simulink model "SystemSimulation"  (R2022a)
settings: Solver=VariableStepAuto  StartTime=0.0  StopTime=Tsim  RelTol=1e-3
values from neighbouring files (symbols this model uses):
  b = 0.0686    [epsac_elbow.m]    (also in modelFinder.m)
  g = 0.8234    [epsac_elbow.m]    (also in modelFinder.m)
  h = 0.3632    [epsac_elbow.m]    (also in modelFinder.m)
  Jeq = 5.4579e-4    (= 0.00054579)    [epsac_elbow.m]    (also in modelFinder.m)
  k = -0.0056    [epsac_elbow.m]    (also in modelFinder.m)
  M = 0.0857    [epsac_elbow.m]    (also in modelFinder.m)
  m = 0.2853    [epsac_elbow.m]    (also in modelFinder.m)
  x = x - x(1)    [modelFinder.m]
settings Model: Creator=aaron  LastModifiedBy=aaron

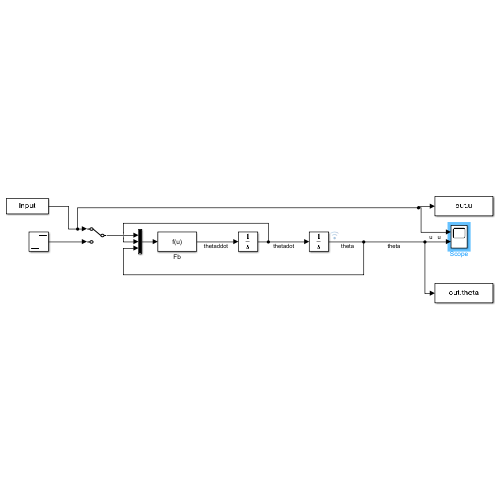
[thumbnail: Simulink's stored preview of the top-level diagram]
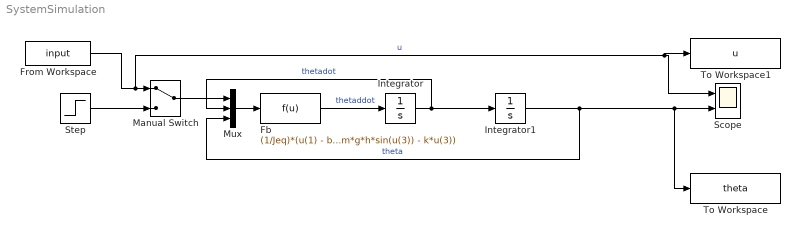
== system SystemSimulation ==
  Fb : Fcn  Expr=(1/Jeq)*(u(1) - b*u(2) - M*g*h*sin(u(3)) - 0.5*m*g*h*sin(u(3)) - k*u(3))
  From Workspace : FromWorkspace  VariableName=input
  Integrator : Integrator
  Integrator1 : Integrator  InitialCondition=x(1)
  Manual Switch : ManualSwitch
  Mux : Mux  Inputs=3
  Scope : Scope  NumInputPorts=2
  Step : Step  SampleTime=0
  To Workspace : ToWorkspace  VariableName=theta  SampleTime=-1
  To Workspace1 : ToWorkspace  VariableName=u  SampleTime=-1
  wires:
  Step/1 -> Manual Switch/2
  Manual Switch/1 -> Mux/1
  Fb/1 -> Integrator/1  "thetaddot"
  Integrator1/1 -> To Workspace/1, Scope/2, Mux/3  "theta"
  Mux/1 -> Fb/1
  From Workspace/1 -> To Workspace1/1, Scope/1, Manual Switch/1  "u"
  Integrator/1 -> Mux/2, Integrator1/1  "thetadot"
